simulink model "kaffeeautomat"  (R2015b)
settings: Solver=FixedStepAuto  StartTime=0.0  StopTime=60  RelTol=1e-3
libraries: simulink x1
settings Model: Creator=scco1019  LastModifiedBy=scco1019

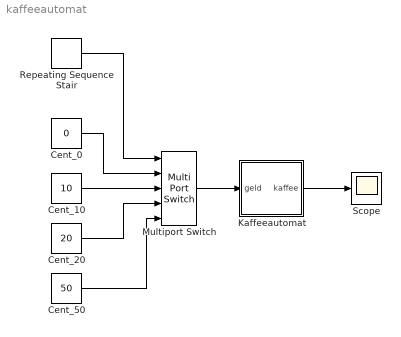
== system kaffeeautomat ==
  Cent_0 : Constant  Value=0
  Cent_10 : Constant  Value=10
  Cent_20 : Constant  Value=20
  Cent_50 : Constant  Value=50
  Kaffeeautomat : Stateflow chart  TreatAsAtomicUnit=on
  Multiport Switch : MultiPortSwitch  Inputs=4
  Repeating Sequence Stair : simulink/Sources/Repeating Sequence Stair  OutValues=[1 2 2 2 2 2 1 2 3 3 1 4 1 2 2 3 3 1 2 2 1 1 1 1 4 1].'  tsamp=-1  OutMin=[]  OutMax=[]  OutDataTypeStr=double  OutputDataTypeScalingMode=double  OutDataType=fixdt(0,8)  ConRadixGroup=Best Precision: Vector-wise  OutScaling=2^-12
  Scope : Scope
  wires:
  Multiport Switch/1 -> Kaffeeautomat/1(geld)
  Repeating Sequence Stair/1 -> Multiport Switch/1
  Cent_0/1 -> Multiport Switch/2
  Cent_10/1 -> Multiport Switch/3
  Cent_20/1 -> Multiport Switch/4
  Cent_50/1 -> Multiport Switch/5
  Kaffeeautomat/1(kaffee) -> Scope/1

== stateflow chart kaffeeautomat/Kaffeeautomat ==
  state CENT_0/
    entry: kaffee=0;
  state CENT_10/
  state CENT_20/
  state CENT_30/
  state CENT_40/
  state CENT_50_PLUS/
    entry: kaffee=1;
  (default) -> CENT_0
  CENT_50_PLUS -> CENT_0
  CENT_0 -> CENT_50_PLUS [order 3] : [geld==50]
  CENT_0 -> CENT_20 [order 1] : [geld==20]
  CENT_0 -> CENT_10 [order 2] : [geld==10]
  CENT_10 -> CENT_30 [order 1] : [geld==20]
  CENT_10 -> CENT_50_PLUS [order 3] : [geld==50]
  CENT_10 -> CENT_20 [order 2] : [geld==10]
  CENT_20 -> CENT_40 [order 1] : [geld==20]
  CENT_20 -> CENT_50_PLUS [order 3] : [geld==50]
  CENT_20 -> CENT_30 [order 2] : [geld==10]
  CENT_30 -> CENT_50_PLUS [order 1] : [geld>=20]
  CENT_30 -> CENT_40 [order 2] : [geld==10]
  CENT_40 -> CENT_50_PLUS : [geld==10]
  data: geld input; kaffee output
